simulink model "Pendulum3DOF"  (R2017a)
settings: Solver=ode45  StartTime=0.0  StopTime=10  MaxStep=0.01  RelTol=1e-3
settings Model: Creator=Charlie  LastModifiedBy=Charlie

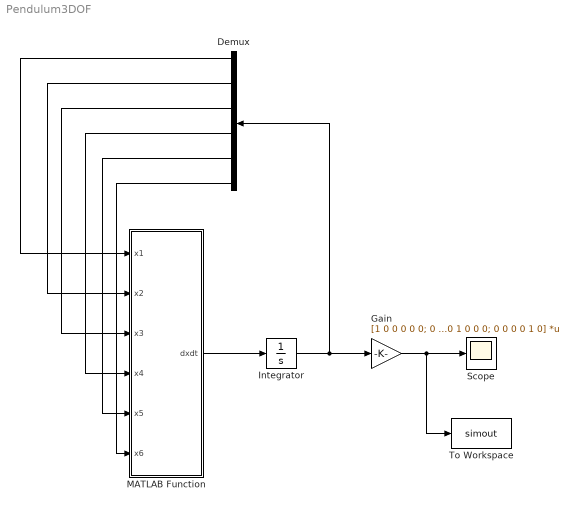
== system Pendulum3DOF ==
  Demux : Demux  Outputs=6
  Gain : Gain  Gain=[1 0 0 0 0 0; 0 0 1 0 0 0; 0 0 0 0 1 0]  Multiplication=Matrix(K*u)
  Integrator : Integrator  InitialCondition=[pi-0.5;0;pi-0.2;0;pi;0]
  MATLAB Function : MATLAB Function  TreatAsAtomicUnit=on
  Scope : Scope
  To Workspace : ToWorkspace  VariableName=simout  SaveFormat=Timeseries  SampleTime=-1
  wires:
  MATLAB Function/1(dxdt) -> Integrator/1
  Integrator/1 -> Demux/1, Gain/1
  Gain/1 -> To Workspace/1, Scope/1
  Demux/6 -> MATLAB Function/6(x6)
  Demux/5 -> MATLAB Function/5(x5)
  Demux/4 -> MATLAB Function/4(x4)
  Demux/3 -> MATLAB Function/3(x3)
  Demux/2 -> MATLAB Function/2(x2)
  Demux/1 -> MATLAB Function/1(x1)

== matlab function Pendulum3DOF/MATLAB Function ==
  data: x1 input; dxdt output; x2 input; x3 input; x4 input; x5 input; x6 input
%function dxdt = dynamics(K,x)
function dxdt = dynamics(x1,x2,x3,x4,x5,x6)

%{
dxdt = [x2;
        -(7*cos(x3)*((981*sin(x1))/100 - (7*x2*x4*sin(x3))/10))/(10*((49*cos(x3)^2)/200 + 1/10000));
        x4;
        -(7000*sin(x3)*((7*cos(x3)*x2^2)/20 + (981*cos(x1))/100))/2451;
        x6;
        0]
%}

% New most accurate
%
dxdt = [x2;
        -((473823*cos(x3)*sin(x1))/2000000000 + (49*x4^2*sin(2*x1))/40000000 + (2401*x4^2*cos(x1)^3*sin(x1))/400000 + (336483*cos(x1)^2*cos(x3)*sin(x1))/2000000 - (2401*x2*x4*sin(2*x3))/400000000 - (336483*cos(x1)^2*cos(x3)^3*sin(x1))/2000000000 + (2401*x4^2*cos(x1)*cos(x3)^2*sin(x1))/400000000 - (3381*x6^2*cos(x1)*cos(x3)^2*sin(x1))/400000000 - (49*x4*x6*cos(x1)^2*cos(x3))/10000000 - (2401*x4*x6*cos(x1)^4*cos(x3))/200000 - (2401*x4^2*cos(x1)^3*cos(x3)^2*sin(x1))/400000000 - (2401*x6^2*cos(x1)^3*cos(x3)^2*sin(x1))/400000 + (2401*x6^2*cos(x1)^3*cos(x3)^4*sin(x1))/400000000 - (2401*x4*x6*cos(x1)^2*cos(x3)^3)/200000000 + (2401*x4*x6*cos(x1)^4*cos(x3)^3)/200000000 + (2401*x2*x4*cos(x1)^2*cos(x3)*sin(x3))/200000000 + (2401*x2*x6*cos(x1)*cos(x3)^2*sin(x1)*sin(x3))/200000000)/((2404381*cos(x1)^2)/400000000 + (2401*cos(x3)^2)/400000000 - (240149*cos(x1)^2*cos(x3)^2)/20000000000 + 49069/20000000000);
        x4;
        (7*cos(x1)*((343483*x2*x4*sin(x1))/20000000 - (48136689*sin(x3))/200000000 + (48069*cos(x1)^2*cos(x3)^2*sin(x3))/200000000 - (343483*x2*x6*cos(x1)*cos(x3))/20000000 + (343*x4^2*cos(x1)^3*cos(x3)*sin(x3))/40000000 + (343*x2*x6*cos(x1)*cos(x3)^3)/20000000 - (343*x2*x4*cos(x3)^2*sin(x1))/20000000 - (343*x6^2*cos(x1)^3*cos(x3)^3*sin(x3))/40000000 - (343*x4^2*cos(x1)*cos(x3)*sin(x3))/40000000 + (343483*x6^2*cos(x1)*cos(x3)*sin(x3))/40000000 + (343*x4*x6*cos(x1)^2*cos(x3)^2*sin(x1)*sin(x3))/20000000))/(10*((2404381*cos(x1)^2)/400000000 + (2401*cos(x3)^2)/400000000 - (240149*cos(x1)^2*cos(x3)^2)/20000000000 + 49069/20000000000));
        x6;
        -(49*((6867*cos(x3)*sin(x1)*sin(x3))/10000000 - (2451*x2*x4*cos(x3))/50000000 - (49*x4^2*cos(x1)^3*sin(x1)*sin(x3))/2000000 - (6867*cos(x1)^2*cos(x3)*sin(x1)*sin(x3))/10000000 + (2451*x2*x4*cos(x1)^2*cos(x3))/50000000 - (x4^2*cos(x1)*sin(x1)*sin(x3))/100000000 - (49*x6^2*cos(x1)*cos(x3)^2*sin(x1)*sin(x3))/2000000 + (2451*x2*x6*cos(x1)*cos(x3)^2*sin(x1))/50000000 + (x4*x6*cos(x1)^2*cos(x3)*sin(x3))/50000000 + (49*x4*x6*cos(x1)^4*cos(x3)*sin(x3))/1000000 + (49*x6^2*cos(x1)^3*cos(x3)^2*sin(x1)*sin(x3))/2000000))/(200*((2404381*cos(x1)^2)/400000000 + (2401*cos(x3)^2)/400000000 - (240149*cos(x1)^2*cos(x3)^2)/20000000000 + 49069/20000000000))]
%}

%{
% As accurate as below 
dxdt = [x2;
        -((473823*cos(x3)*sin(x1))/2000000000 + (49*x4^2*sin(2*x1))/40000000 + (2401*x4^2*cos(x1)^3*sin(x1))/400000 + (336483*cos(x1)^2*cos(x3)*sin(x1))/2000000 - (2401*x2*x4*sin(2*x3))/400000000 - (336483*cos(x1)^2*cos(x3)^3*sin(x1))/2000000000 + (2401*x4^2*cos(x1)*cos(x3)^2*sin(x1))/400000000 - (3381*x6^2*cos(x1)*cos(x3)^2*sin(x1))/400000000 + (49*x4*x6*cos(x1)^2*cos(x3))/10000000 + (2401*x4*x6*cos(x1)^4*cos(x3))/200000 - (2401*x4^2*cos(x1)^3*cos(x3)^2*sin(x1))/400000000 - (2401*x6^2*cos(x1)^3*cos(x3)^2*sin(x1))/400000 + (2401*x6^2*cos(x1)^3*cos(x3)^4*sin(x1))/400000000 + (2401*x4*x6*cos(x1)^2*cos(x3)^3)/200000000 - (2401*x4*x6*cos(x1)^4*cos(x3)^3)/200000000 + (2401*x2*x4*cos(x1)^2*cos(x3)*sin(x3))/200000000 - (2401*x2*x6*cos(x1)*cos(x3)^2*sin(x1)*sin(x3))/200000000)/((2404381*cos(x1)^2)/400000000 + (2401*cos(x3)^2)/400000000 - (240149*cos(x1)^2*cos(x3)^2)/20000000000 + 49069/20000000000);
        x4;
        -(7*cos(x1)*((48136689*sin(x3))/200000000 - (343483*x2*x4*sin(x1))/20000000 - (48069*cos(x1)^2*cos(x3)^2*sin(x3))/200000000 - (343483*x2*x6*cos(x1)*cos(x3))/20000000 - (343*x4^2*cos(x1)^3*cos(x3)*sin(x3))/40000000 + (343*x2*x6*cos(x1)*cos(x3)^3)/20000000 + (343*x2*x4*cos(x3)^2*sin(x1))/20000000 + (343*x6^2*cos(x1)^3*cos(x3)^3*sin(x3))/40000000 + (343*x4^2*cos(x1)*cos(x3)*sin(x3))/40000000 - (343483*x6^2*cos(x1)*cos(x3)*sin(x3))/40000000 + (343*x4*x6*cos(x1)^2*cos(x3)^2*sin(x1)*sin(x3))/20000000))/(10*((2404381*cos(x1)^2)/400000000 + (2401*cos(x3)^2)/400000000 - (240149*cos(x1)^2*cos(x3)^2)/20000000000 + 49069/20000000000));
        x6;
        -(49*((2451*x2*x4*cos(x3))/50000000 - (6867*cos(x3)*sin(x1)*sin(x3))/10000000 + (49*x4^2*cos(x1)^3*sin(x1)*sin(x3))/2000000 + (6867*cos(x1)^2*cos(x3)*sin(x1)*sin(x3))/10000000 - (2451*x2*x4*cos(x1)^2*cos(x3))/50000000 + (x4^2*cos(x1)*sin(x1)*sin(x3))/100000000 + (49*x6^2*cos(x1)*cos(x3)^2*sin(x1)*sin(x3))/2000000 + (2451*x2*x6*cos(x1)*cos(x3)^2*sin(x1))/50000000 + (x4*x6*cos(x1)^2*cos(x3)*sin(x3))/50000000 + (49*x4*x6*cos(x1)^4*cos(x3)*sin(x3))/1000000 - (49*x6^2*cos(x1)^3*cos(x3)^2*sin(x1)*sin(x3))/2000000))/(200*((2404381*cos(x1)^2)/400000000 + (2401*cos(x3)^2)/400000000 - (240149*cos(x1)^2*cos(x3)^2)/20000000000 + 49069/20000000000))]
%}

%{
% Most accurate so far
dxdt = [x2;
        -((350217*cos(x3)*sin(x1))/2000000000 + (49*x4^2*sin(2*x1))/400000000 + (2401*x4^2*cos(x1)^3*sin(x1))/4000000 + (336483*cos(x1)^2*cos(x3)*sin(x1))/20000000 - (2401*x2*x4*sin(2*x3))/400000000 - (336483*cos(x1)^2*cos(x3)^3*sin(x1))/2000000000 + (2401*x4^2*cos(x1)*cos(x3)^2*sin(x1))/400000000 - (2499*x6^2*cos(x1)*cos(x3)^2*sin(x1))/400000000 + (49*x4*x6*cos(x1)^2*cos(x3))/100000000 + (2401*x4*x6*cos(x1)^4*cos(x3))/2000000 - (2401*x4^2*cos(x1)^3*cos(x3)^2*sin(x1))/400000000 - (2401*x6^2*cos(x1)^3*cos(x3)^2*sin(x1))/4000000 + (2401*x6^2*cos(x1)^3*cos(x3)^4*sin(x1))/400000000 + (2401*x4*x6*cos(x1)^2*cos(x3)^3)/200000000 - (2401*x4*x6*cos(x1)^4*cos(x3)^3)/200000000 + (2401*x2*x4*cos(x1)^2*cos(x3)*sin(x3))/200000000 - (2401*x2*x6*cos(x1)*cos(x3)^2*sin(x1)*sin(x3))/200000000)/((242599*cos(x1)^2)/400000000 + (2401*cos(x3)^2)/400000000 - (240149*cos(x1)^2*cos(x3)^2)/20000000000 + 4951/20000000000);
        x4;
        -(7*cos(x1)*((4856931*sin(x3))/200000000 - (34657*x2*x4*sin(x1))/20000000 - (48069*cos(x1)^2*cos(x3)^2*sin(x3))/200000000 - (34657*x2*x6*cos(x1)*cos(x3))/20000000 - (343*x4^2*cos(x1)^3*cos(x3)*sin(x3))/40000000 + (343*x2*x6*cos(x1)*cos(x3)^3)/20000000 + (343*x2*x4*cos(x3)^2*sin(x1))/20000000 + (343*x6^2*cos(x1)^3*cos(x3)^3*sin(x3))/40000000 + (343*x4^2*cos(x1)*cos(x3)*sin(x3))/40000000 - (34657*x6^2*cos(x1)*cos(x3)*sin(x3))/40000000 + (343*x4*x6*cos(x1)^2*cos(x3)^2*sin(x1)*sin(x3))/20000000))/(10*((242599*cos(x1)^2)/400000000 + (2401*cos(x3)^2)/400000000 - (240149*cos(x1)^2*cos(x3)^2)/20000000000 + 4951/20000000000));
        x6;
        -(49*((2451*x2*x4*cos(x3))/50000000 - (6867*cos(x3)*sin(x1)*sin(x3))/10000000 + (49*x4^2*cos(x1)^3*sin(x1)*sin(x3))/2000000 + (6867*cos(x1)^2*cos(x3)*sin(x1)*sin(x3))/10000000 - (2451*x2*x4*cos(x1)^2*cos(x3))/50000000 + (x4^2*cos(x1)*sin(x1)*sin(x3))/100000000 + (49*x6^2*cos(x1)*cos(x3)^2*sin(x1)*sin(x3))/2000000 + (2451*x2*x6*cos(x1)*cos(x3)^2*sin(x1))/50000000 + (x4*x6*cos(x1)^2*cos(x3)*sin(x3))/50000000 + (49*x4*x6*cos(x1)^4*cos(x3)*sin(x3))/1000000 - (49*x6^2*cos(x1)^3*cos(x3)^2*sin(x1)*sin(x3))/2000000))/(200*((242599*cos(x1)^2)/400000000 + (2401*cos(x3)^2)/400000000 - (240149*cos(x1)^2*cos(x3)^2)/20000000000 + 4951/20000000000))]
%}

%{
% Yaw affects pitch and roll.
dxdt = [x2;
        -(4000000*((2401*x4^2*cos(x1)^3*sin(x1))/4000000 + (336483*cos(x1)^2*cos(x3)*sin(x1))/20000000 + (2401*x4*x6*cos(x1)^4*cos(x3))/2000000 - (2401*x6^2*cos(x1)^3*cos(x3)^2*sin(x1))/4000000))/(2401*cos(x1)^2);
        x4;
        (400000*((343*cos(x1)*cos(x3)*sin(x3)*x6^2)/400000 + (343*x2*cos(x1)*cos(x3)*x6)/200000 - (48069*sin(x3))/2000000 + (343*x2*x4*sin(x1))/200000))/(343*cos(x1));
        x6;
        0]
%}

%{
dxdt = [x2;
        -(7*cos(x3)*((981*sin(x1))/100 - (7*x2*x4*sin(x3))/10))/(10*((49*cos(x3)^2)/200 + 1));
        x4;
        -(140*sin(x3)*((7*cos(x3)*x2^2)/20 + (981*cos(x1))/100))/249;
        x6;
        0.1*x5]
%}

%{
dxdt = [x(2);
        ((1421469*cos(x(3))*sin(x(1)))/400000 - (147*x(4)^2*sin(2*x(1)))/8000 - (2401*x(4)^2*cos(x(1))^3*sin(x(1)))/400000 + (336483*cos(x(1))^2*cos(x(3))*sin(x(1)))/2000000 + (7203*x(2)*x(4)*sin(2*x(3)))/80000 - (1009449*cos(x(1))^2*cos(x(3))^3*sin(x(1)))/400000 - (7203*x(4)^2*cos(x(1))*cos(x(3))^2*sin(x(1)))/80000 + (10143*x(6)^2*cos(x(1))*cos(x(3))^2*sin(x(1)))/80000 + (147*x(4)*x(6)*cos(x(1))^2*cos(x(3)))/2000 + (2401*x(4)*x(6)*cos(x(1))^4*cos(x(3)))/200000 + (7203*x(4)^2*cos(x(1))^3*cos(x(3))^2*sin(x(1)))/80000 + (2401*x(6)^2*cos(x(1))^3*cos(x(3))^2*sin(x(1)))/400000 - (7203*x(6)^2*cos(x(1))^3*cos(x(3))^4*sin(x(1)))/80000 + (7203*x(4)*x(6)*cos(x(1))^2*cos(x(3))^3)/40000 - (7203*x(4)*x(6)*cos(x(1))^4*cos(x(3))^3)/40000 - (7203*x(2)*x(4)*cos(x(1))^2*cos(x(3))*sin(x(3)))/40000 - (7203*x(2)*x(6)*cos(x(1))*cos(x(3))^2*sin(x(1))*sin(x(3)))/40000)/((13279*cos(x(1))^2)/100000 + (7203*cos(x(3))^2)/80000 - (29253*cos(x(1))^2*cos(x(3))^2)/40000 + 813/1000);
        x(4);
        (7*cos(x(1))*((265851*sin(x(3)))/50000 + (1897*x(2)*x(4)*sin(x(1)))/5000 - (144207*cos(x(1))^2*cos(x(3))^2*sin(x(3)))/40000 - (1897*x(2)*x(6)*cos(x(1))*cos(x(3)))/5000 + (1029*x(4)^2*cos(x(1))^3*cos(x(3))*sin(x(3)))/8000 + (1029*x(2)*x(6)*cos(x(1))*cos(x(3))^3)/4000 - (1029*x(2)*x(4)*cos(x(3))^2*sin(x(1)))/4000 - (1029*x(6)^2*cos(x(1))^3*cos(x(3))^3*sin(x(3)))/8000 - (1029*x(4)^2*cos(x(1))*cos(x(3))*sin(x(3)))/8000 + (1897*x(6)^2*cos(x(1))*cos(x(3))*sin(x(3)))/10000 + (1029*x(4)*x(6)*cos(x(1))^2*cos(x(3))^2*sin(x(1))*sin(x(3)))/4000))/(10*((13279*cos(x(1))^2)/100000 + (7203*cos(x(3))^2)/80000 - (29253*cos(x(1))^2*cos(x(3))^2)/40000 + 813/1000));
        x(6);
        -(49*((20601*cos(x(1))^2*cos(x(3))*sin(x(1))*sin(x(3)))/2000 - (1047*x(2)*x(4)*cos(x(3)))/200 - (147*x(4)^2*cos(x(1))^3*sin(x(1))*sin(x(3)))/400 - (20601*cos(x(3))*sin(x(1))*sin(x(3)))/2000 + (1047*x(2)*x(4)*cos(x(1))^2*cos(x(3)))/200 - (9*x(4)^2*cos(x(1))*sin(x(1))*sin(x(3)))/4 - (147*x(6)^2*cos(x(1))*cos(x(3))^2*sin(x(1))*sin(x(3)))/400 + (1047*x(2)*x(6)*cos(x(1))*cos(x(3))^2*sin(x(1)))/200 + (9*x(4)*x(6)*cos(x(1))^2*cos(x(3))*sin(x(3)))/2 + (147*x(4)*x(6)*cos(x(1))^4*cos(x(3))*sin(x(3)))/200 + (147*x(6)^2*cos(x(1))^3*cos(x(3))^2*sin(x(1))*sin(x(3)))/400))/(200*((13279*cos(x(1))^2)/100000 + (7203*cos(x(3))^2)/80000 - (29253*cos(x(1))^2*cos(x(3))^2)/40000 + 813/1000));
       ]
%}
